simulink model "MySimModel"  (R2024b)
settings: Solver=VariableStepAuto  StartTime=0.0  StopTime=10.0  RelTol=1e-3
settings Model: Creator=xinxing  LastModifiedBy=xinxing

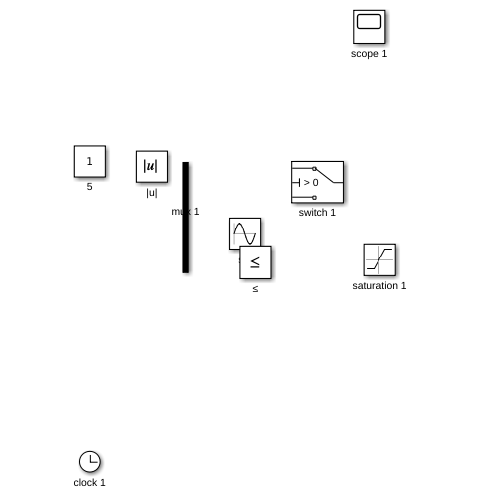
[thumbnail: Simulink's stored preview of the top-level diagram]
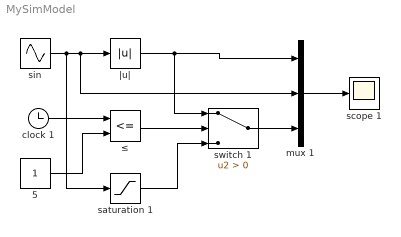
== system MySimModel ==
  5 : Constant
  clock 1 : Clock
  mux 1 : Mux  Inputs=3
  saturation 1 : Saturate
  scope 1 : Scope
  sin : Sin  SampleTime=0
  switch 1 : Switch  Criteria=u2 > Threshold  SaturateOnIntegerOverflow=off  InputSameDT=off
  |u| : Abs  SaturateOnIntegerOverflow=off
  ≤ : RelationalOperator  Operator=<=  OutDataTypeStr=boolean  RndMeth=Simplest  InputSameDT=off
  wires:
  mux 1/1 -> scope 1/1
  switch 1/1 -> mux 1/3
  saturation 1/1 -> switch 1/3
  ≤/1 -> switch 1/2
  |u|/1 -> switch 1/1, mux 1/1
  5/1 -> ≤/2
  clock 1/1 -> ≤/1
  sin/1 -> |u|/1, mux 1/2, saturation 1/1
